simulink model "Roboter_RRP_Sim"  (R2015b)
settings: Solver=ode15s  StartTime=0.0  StopTime=5  RelTol=1e-6  AbsTol=1e-5
InitFcn:
  | set_parameter
StartFcn:
  | set_parameter
StopFcn:
  | Auswertung
undefined symbols (not defined in the file or in its folder): parReg, parSys
settings Model: Creator=andreas  LastModifiedBy=Andreas
settings SolverCC: MaxOrder=3
settings DataIOCC: SaveFormat=Array  SignalLoggingSaveFormat=ModelDataLogs
settings OptimizationCC: ExpressionDepthLimit=2147483647  InitFltsAndDblsToZero=on
settings DebuggingCC: SaveWithParameterizedLinksMsg=none  UnderspecifiedInitializationDetection=Classic  MergeDetectMultiDrivingBlocksExec=none  SignalResolutionControl=TryResolveAllWithWarning  SolverPrmCheckMsg=warning  MultiTaskDSMMsg=warning  MultiTaskCondExecSysMsg=none  FcnCallInpInsideContextMsg=UseLocalSettings  StateNameClashWarn=warning
settings HardwareCC: ProdBitPerPointer=32  ProdLargestAtomicFloat=None  ProdIntDivRoundTo=Undefined  ProdEndianess=Unspecified  ProdWordSize=32  ProdHWDeviceType=32-bit Generic
settings GRTTargetCC: TargetFcnLib=ansi_tfl_tmw.mat  GeneratePreprocessorConditionals=Disable all  CombineOutputUpdateFcns=off  GRTInterface=on
settings ConfigComp: CovModelRefEnable=Off

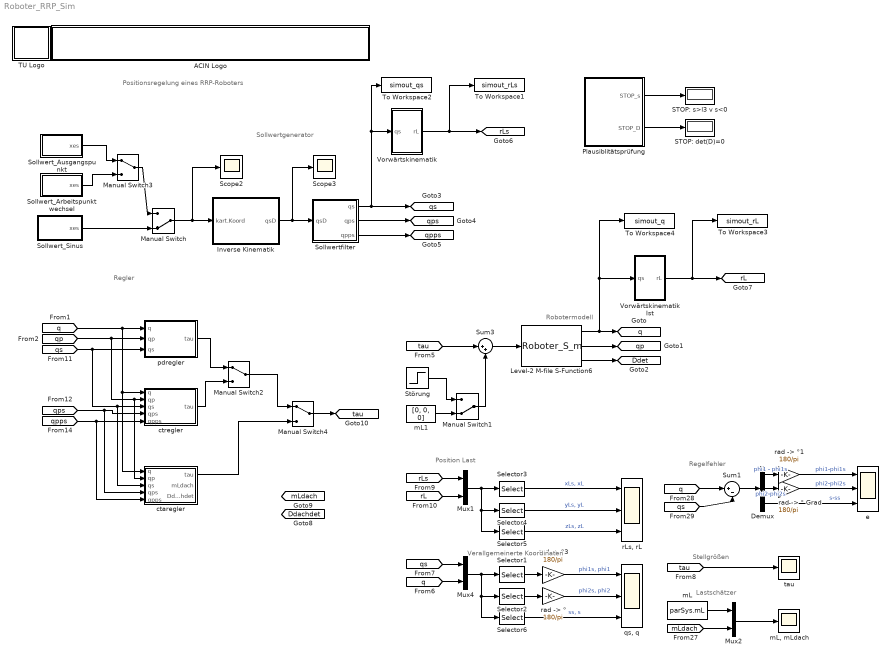
== system Roboter_RRP_Sim ==
  note: Positionsregelung eines RRP-Roboters
  note: Robotermodell
  note: Regler
  note: Sollwertgenerator
  note: Position Last
  note: Verallgemeinerte Koordinaten
  note: Regelfehler
  note: Stellgrößen
  note: Lastschätzer
  ACIN Logo : Subsystem
      mask init:
      | s = get_param(gcb,'UserData');
      mask Display:
      | image(s.logo,[0 0 439 45]);
      | %axis image
  Demux : Demux  Outputs=3
  Inverse Kinematik : Subsystem
  Level-2 M-file S-Function6 : M-S-Function  FunctionName=Roboter_S_m  Parameters=m1,m2,m3,mL,l1,l2,l3,Ixx1,Iyy1,Izz1,Ixx2,Iyy2,Izz2,Ixx3,Iyy3,Izz3,d1,d2,d3,phi10,phi20,s0  mask{m1=parSys.m1, m2=parSys.m2, m3=parSys.m3, mL=parSys.mL, l1=parSys.l1, l2=parSys.l2, l3=parSys.l3, Ixx1=parSys.Ixx1, Iyy1=parSys.Iyy1, Izz1=parSys.Izz1, Ixx2=parSys.Ixx2, Iyy2=parSys.Iyy2, Izz2=parSys.Izz2, Ixx3=parSys.Ixx3, Iyy3=parSys.Iyy3, Izz3=parSys.Izz3, d1=parSys.d1, d2=parSys.d2, d3=parSys.d3, phi10=parSys.phi10, phi20=parSys.phi20, s0=parSys.s0}
      mask prompts: m1 "Masse Stab 1"; m2 "Masse Stab 2"; m3 "Masse Stab 3"; mL "Masse Last"; l1 "Länge Stab 1"; l2 "Länge Stab 2"; l3 "Länge Stab 3"; Ixx1 "Trägheitsmoment x Stab 1"; Iyy1 "Trägheitsmoment y Stab 1"; Izz1 "Trägheitsmoment z Stab 1"; Ixx2 "Trägheitsmoment x Stab 2"; Iyy2 "Trägheitsmoment y Stab 2"; Izz2 "Trägheitsmoment z Stab 2"; Ixx3 "Trägheitsmoment x Stab 3"; Iyy3 "Trägheitsmoment y Stab 3"; Izz3 "Trägheitsmoment z Stab 3"; d1 "Dämpfung Stab 1"; d2 "Dämpfung Stab 2"; d3 "Dämpfung Stab 3"; phi10 "AB phi1"; phi20 "AB phi2"; s0 "AB s"
  Manual Switch : ManualSwitch  CurrentSetting=0
  Manual Switch1 : ManualSwitch  CurrentSetting=0
  Manual Switch2 : ManualSwitch
  Manual Switch3 : ManualSwitch
  Manual Switch4 : ManualSwitch
  Mux1 : Mux  Inputs=2
  Mux2 : Mux  Inputs=2
  Mux4 : Mux  Inputs=2
  Plausiblitätsprüfung : Subsystem
  STOP: det(D)=0 : Display
  STOP: s>l3 v s<0 : Display
  Scope2 : Scope
  Scope3 : Scope
  Selector1 : Selector  InputPortWidth=6  IndexOptions=Index vector (dialog)  Indices=[1 4]  OutputSizes=1
  Selector2 : Selector  InputPortWidth=6  IndexOptions=Index vector (dialog)  Indices=[2 5]  OutputSizes=1
  Selector3 : Selector  InputPortWidth=6  IndexOptions=Index vector (dialog)  Indices=[1 4]  OutputSizes=1
  Selector4 : Selector  InputPortWidth=6  IndexOptions=Index vector (dialog)  Indices=[2 5]  OutputSizes=1
  Selector5 : Selector  InputPortWidth=6  IndexOptions=Index vector (dialog)  Indices=[3 6]  OutputSizes=1
  Selector6 : Selector  InputPortWidth=6  IndexOptions=Index vector (dialog)  Indices=[3 6]  OutputSizes=1
  Sollwert_Arbeitspunktwechsel : Subsystem
  Sollwert_Ausgangspunkt : Subsystem
  Sollwert_Sinus : Subsystem
  Sollwertfilter : Subsystem
  Störung : Step  After=[300, 300, 200]  SampleTime=0
  Sum1 : Sum  Inputs=|+-
  Sum3 : Sum  Inputs=|++
  TU Logo : Subsystem
      mask init:
      | s = get_param(gcb,'UserData');
      mask Display: image(s.logo,[0 0 45 45]);
  To Workspace1 : ToWorkspace  VariableName=simout_rLs  SaveFormat=Structure With Time  SampleTime=-1
  To Workspace2 : ToWorkspace  VariableName=simout_qs  SaveFormat=Structure With Time  SampleTime=-1
  To Workspace3 : ToWorkspace  VariableName=simout_rL  SaveFormat=Structure With Time  SampleTime=-1
  To Workspace4 : ToWorkspace  VariableName=simout_q  SaveFormat=Structure With Time  SampleTime=-1
  Vorwärtskinematik : Subsystem
  Vorwärtskinematik Ist : Subsystem
  ctaregler : MATLAB Function  TreatAsAtomicUnit=on
  ctregler : MATLAB Function  TreatAsAtomicUnit=on
  e : Scope  NumInputPorts=3
  mL : Constant  Value=parSys.mL
  "mL, mLdach" : Scope
  mL1 : Constant  Value=[0, 0, 0]
  pdregler : MATLAB Function  TreatAsAtomicUnit=on
  "qs, q" : Scope  NumInputPorts=3
  "rLs, rL" : Scope  NumInputPorts=3
  "rad -> °" : Gain  Gain=180/pi
  "rad -> ° Grad" : Gain  Gain=180/pi
  "rad -> °1" : Gain  Gain=180/pi
  "rad -> °3" : Gain  Gain=180/pi
  tau : Scope
  tag scope: Ddachdet=global, Ddet=global, mLdach=global, q=global, qp=global, qpps=global, qps=global, qs=global, rL=global, rLs=global, tau=global
  wires:
  Level-2 M-file S-Function6/1 -> [q], Vorwärtskinematik Ist/1(qs), To Workspace4/1
  Level-2 M-file S-Function6/2 -> [qp]
  Inverse Kinematik/1(qsD) -> Scope3/1, Sollwertfilter/1(qsD)
  [tau] -> tau/1
  Vorwärtskinematik Ist/1(rL) -> [rL], To Workspace3/1
  Manual Switch/1 -> Inverse Kinematik/1(kart.Koord), Scope2/1
  Sollwert_Sinus/1(xes) -> Manual Switch/2
  [qs] -> Mux4/1
  [q] -> Mux4/2
  Mux4/1 -> Selector1/1, Selector2/1, Selector6/1
  [rLs] -> Mux1/1
  [rL] -> Mux1/2
  Selector3/1 -> "rLs, rL"/1  "xLs, xL"
  Selector4/1 -> "rLs, rL"/2  "yLs, yL"
  Selector5/1 -> "rLs, rL"/3  "zLs, zL"
  Mux1/1 -> Selector5/1, Selector4/1, Selector3/1
  Manual Switch3/1 -> Manual Switch/1
  Sollwert_Arbeitspunktwechsel/1(xes) -> Manual Switch3/2
  Sollwert_Ausgangspunkt/1(xes) -> Manual Switch3/1
  Plausiblitätsprüfung/1(STOP_s) -> STOP: s>l3 v s<0/1
  Sollwertfilter/1(qs) -> [qs], Vorwärtskinematik/1(qs), To Workspace2/1
  Sollwertfilter/3(qpps) -> [qpps]
  Sollwertfilter/2(qps) -> [qps]
  [q] -> Sum1/1
  Demux/1 -> "rad -> °1"/1  "phi1 - phi1s"
  Demux/2 -> "rad -> ° Grad"/1  "phi2-phi2s"
  Demux/3 -> e/3  "s-ss"
  [qs] -> Sum1/2
  Sum1/1 -> Demux/1
  [tau] -> Sum3/1
  Sum3/1 -> Level-2 M-file S-Function6/1
  Störung/1 -> Manual Switch1/1
  mL1/1 -> Manual Switch1/2
  Manual Switch1/1 -> Sum3/2
  Mux2/1 -> "mL, mLdach"/1
  mL/1 -> Mux2/1
  [mLdach] -> Mux2/2
  Selector1/1 -> "rad -> °3"/1
  Selector2/1 -> "rad -> °"/1
  Selector6/1 -> "qs, q"/3  "ss, s"
  "rad -> °"/1 -> "qs, q"/2  "phi2s, phi2"
  "rad -> °3"/1 -> "qs, q"/1  "phi1s, phi1"
  "rad -> °1"/1 -> e/1  "phi1-phi1s"
  "rad -> ° Grad"/1 -> e/2  "phi2-phi2s"
  Vorwärtskinematik/1(rL) -> [rLs], To Workspace1/1
  Plausiblitätsprüfung/2(STOP_D) -> STOP: det(D)=0/1
  Level-2 M-file S-Function6/3 -> [Ddet]
  [q] -> ctaregler/1(q), ctregler/1(q), pdregler/1(q)
  [qs] -> ctaregler/3(qs), ctregler/3(qs), pdregler/3(qs)
  pdregler/1(tau) -> Manual Switch2/1
  ctregler/1(tau) -> Manual Switch2/2
  [qpps] -> ctaregler/5(qpps), ctregler/5(qpps)
  [qps] -> ctaregler/4(qps), ctregler/4(qps)
  [qp] -> ctaregler/2(qp), ctregler/2(qp), pdregler/2(qp)
  Manual Switch4/1 -> [tau]
  Manual Switch2/1 -> Manual Switch4/1
  ctaregler/1(tau) -> Manual Switch4/2

== system Roboter_RRP_Sim/ACIN Logo ==

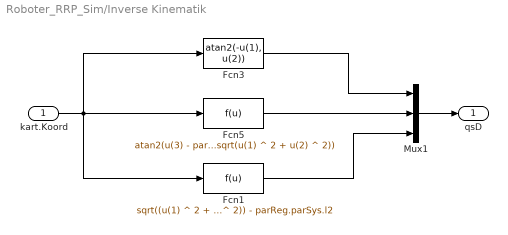
== system Roboter_RRP_Sim/Inverse Kinematik ==
  kart.Koord : Inport
  Fcn1 : Fcn  Expr=sqrt((u(1) ^ 2 + u(2) ^ 2 + u(3) ^ 2 - 2 * u(3) * parReg.parSys.l1 + parReg.parSys.l1 ^ 2)) - parReg.parSys.l2
  Fcn3 : Fcn  Expr=atan2(-u(1), u(2))
  Fcn5 : Fcn  Expr=atan2(u(3) - parReg.parSys.l1, sqrt(u(1) ^ 2 + u(2) ^ 2))
  Mux1 : Mux  Inputs=3
  qsD : Outport
  wires:
  kart.Koord/1 -> Fcn3/1, Fcn1/1, Fcn5/1
  Fcn3/1 -> Mux1/1
  Fcn5/1 -> Mux1/2
  Mux1/1 -> qsD/1
  Fcn1/1 -> Mux1/3

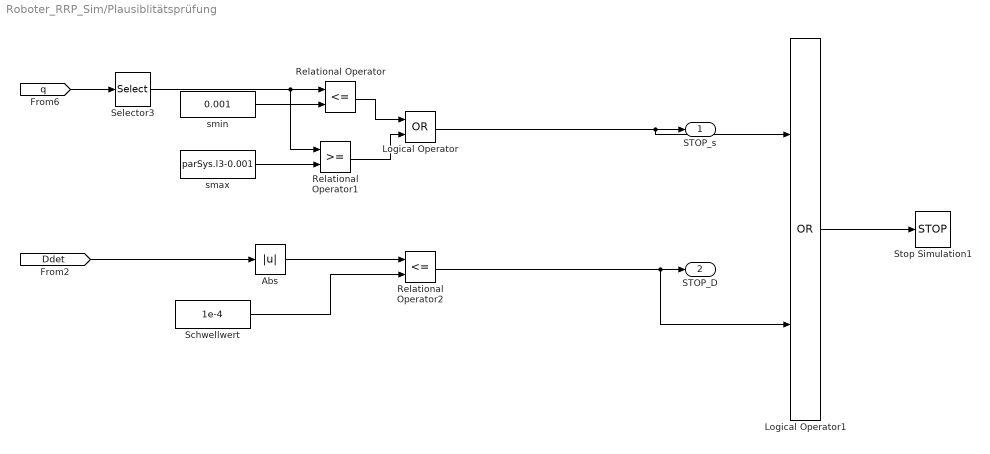
== system Roboter_RRP_Sim/Plausiblitätsprüfung ==
  Abs : Abs
  Logical Operator : Logic  Operator=OR  AllPortsSameDT=off  OutDataTypeStr=boolean
  Logical Operator1 : Logic  Operator=OR  AllPortsSameDT=off  OutDataTypeStr=boolean
  Relational Operator : RelationalOperator  Operator=<=  OutDataTypeStr=boolean
  Relational Operator1 : RelationalOperator  OutDataTypeStr=boolean
  Relational Operator2 : RelationalOperator  Operator=<=  OutDataTypeStr=boolean
  Schwellwert : Constant  Value=1e-4
  Selector3 : Selector  InputPortWidth=3  IndexOptions=Index vector (dialog)  Indices=[3]  OutputSizes=1
  Stop Simulation1 : Stop
  smax : Constant  Value=parSys.l3-0.001
  smin : Constant  Value=0.001
  STOP_s : Outport
  STOP_D : Outport  Port=2
  wires:
  Relational Operator/1 -> Logical Operator/1
  Relational Operator1/1 -> Logical Operator/2
  [q] -> Selector3/1
  Selector3/1 -> Relational Operator/1, Relational Operator1/1
  smin/1 -> Relational Operator/2
  [Ddet] -> Abs/1
  Abs/1 -> Relational Operator2/1
  Schwellwert/1 -> Relational Operator2/2
  Logical Operator1/1 -> Stop Simulation1/1
  smax/1 -> Relational Operator1/2
  Relational Operator2/1 -> STOP_D/1, Logical Operator1/2
  Logical Operator/1 -> STOP_s/1, Logical Operator1/1

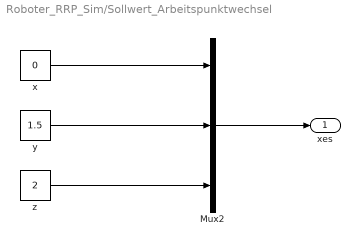
== system Roboter_RRP_Sim/Sollwert_Arbeitspunktwechsel ==
  Mux2 : Mux  Inputs=3
  x : Constant  Value=0
  y : Constant  Value=1.5
  z : Constant  Value=2
  xes : Outport
  wires:
  Mux2/1 -> xes/1
  x/1 -> Mux2/1
  y/1 -> Mux2/2
  z/1 -> Mux2/3

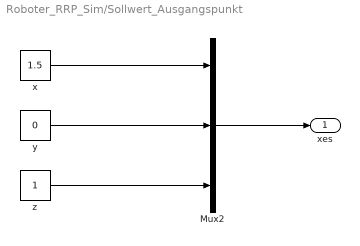
== system Roboter_RRP_Sim/Sollwert_Ausgangspunkt ==
  Mux2 : Mux  Inputs=3
  x : Constant  Value=1.5
  y : Constant  Value=0
  z : Constant
  xes : Outport
  wires:
  z/1 -> Mux2/3
  y/1 -> Mux2/2
  x/1 -> Mux2/1
  Mux2/1 -> xes/1

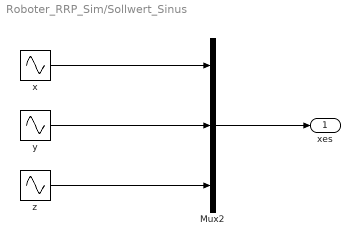
== system Roboter_RRP_Sim/Sollwert_Sinus ==
  Mux2 : Mux  Inputs=3
  x : Sin  Amplitude=1.5  Frequency=2*pi*parReg.traj_fKreis  Phase=pi/2  SampleTime=0
  y : Sin  Amplitude=1.5  Frequency=2*pi*parReg.traj_fKreis  SampleTime=0
  z : Sin  Amplitude=0.5  Bias=1.5  Frequency=2*pi*parReg.traj_fz  Phase=-pi/2  SampleTime=0
  xes : Outport
  wires:
  Mux2/1 -> xes/1
  x/1 -> Mux2/1
  y/1 -> Mux2/2
  z/1 -> Mux2/3

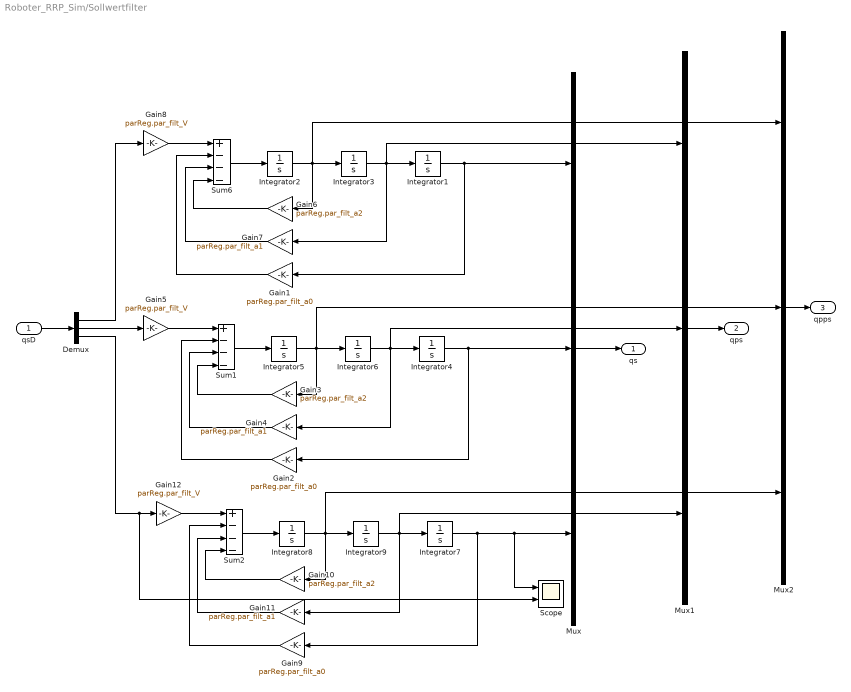
== system Roboter_RRP_Sim/Sollwertfilter ==
  qsD : Inport
  Demux : Demux  Outputs=3
  Gain1 : Gain  Gain=parReg.par_filt_a0  SaturateOnIntegerOverflow=on  OutDataTypeStr=Inherit: Same as input  ParamDataTypeStr=Inherit: Same as input
  Gain10 : Gain  Gain=parReg.par_filt_a2  SaturateOnIntegerOverflow=on  OutDataTypeStr=Inherit: Same as input  ParamDataTypeStr=Inherit: Same as input
  Gain11 : Gain  Gain=parReg.par_filt_a1  SaturateOnIntegerOverflow=on  OutDataTypeStr=Inherit: Same as input  ParamDataTypeStr=Inherit: Same as input
  Gain12 : Gain  Gain=parReg.par_filt_V  SaturateOnIntegerOverflow=on  OutDataTypeStr=Inherit: Same as input  ParamDataTypeStr=Inherit: Same as input
  Gain2 : Gain  Gain=parReg.par_filt_a0  SaturateOnIntegerOverflow=on  OutDataTypeStr=Inherit: Same as input  ParamDataTypeStr=Inherit: Same as input
  Gain3 : Gain  Gain=parReg.par_filt_a2  SaturateOnIntegerOverflow=on  OutDataTypeStr=Inherit: Same as input  ParamDataTypeStr=Inherit: Same as input
  Gain4 : Gain  Gain=parReg.par_filt_a1  SaturateOnIntegerOverflow=on  OutDataTypeStr=Inherit: Same as input  ParamDataTypeStr=Inherit: Same as input
  Gain5 : Gain  Gain=parReg.par_filt_V  SaturateOnIntegerOverflow=on  OutDataTypeStr=Inherit: Same as input  ParamDataTypeStr=Inherit: Same as input
  Gain6 : Gain  Gain=parReg.par_filt_a2  SaturateOnIntegerOverflow=on  OutDataTypeStr=Inherit: Same as input  ParamDataTypeStr=Inherit: Same as input
  Gain7 : Gain  Gain=parReg.par_filt_a1  SaturateOnIntegerOverflow=on  OutDataTypeStr=Inherit: Same as input  ParamDataTypeStr=Inherit: Same as input
  Gain8 : Gain  Gain=parReg.par_filt_V  SaturateOnIntegerOverflow=on  OutDataTypeStr=Inherit: Same as input  ParamDataTypeStr=Inherit: Same as input
  Gain9 : Gain  Gain=parReg.par_filt_a0  SaturateOnIntegerOverflow=on  OutDataTypeStr=Inherit: Same as input  ParamDataTypeStr=Inherit: Same as input
  Integrator1 : Integrator  InitialCondition=parReg.traj_phi10
  Integrator{2..3,5..6,8..9} (6 alike) : Integrator
  Integrator4 : Integrator  InitialCondition=parReg.traj_phi20
  Integrator7 : Integrator  InitialCondition=parReg.traj_s0
  Mux : Mux  Inputs=3
  Mux1 : Mux  Inputs=3
  Mux2 : Mux  Inputs=3
  Scope : Scope  NumInputPorts=2
  Sum1 : Sum  Inputs=+---  SaturateOnIntegerOverflow=on  InputSameDT=on  OutDataTypeStr=Inherit: Same as first input
  Sum2 : Sum  Inputs=+---  SaturateOnIntegerOverflow=on  InputSameDT=on  OutDataTypeStr=Inherit: Same as first input
  Sum6 : Sum  Inputs=+---  SaturateOnIntegerOverflow=on  InputSameDT=on  OutDataTypeStr=Inherit: Same as first input
  qs : Outport
  qps : Outport  Port=2
  qpps : Outport  Port=3
  wires:
  Mux/1 -> qs/1
  qsD/1 -> Demux/1
  Demux/1 -> Gain8/1
  Sum6/1 -> Integrator2/1
  Gain8/1 -> Sum6/1
  Integrator3/1 -> Integrator1/1, Gain7/1, Mux1/1
  Integrator2/1 -> Integrator3/1, Gain6/1, Mux2/1
  Integrator1/1 -> Gain1/1, Mux/1
  Gain6/1 -> Sum6/4
  Gain7/1 -> Sum6/3
  Gain1/1 -> Sum6/2
  Sum1/1 -> Integrator5/1
  Gain5/1 -> Sum1/1
  Integrator6/1 -> Gain4/1, Integrator4/1, Mux1/2
  Integrator5/1 -> Gain3/1, Integrator6/1, Mux2/2
  Integrator4/1 -> Gain2/1, Mux/2
  Gain3/1 -> Sum1/4
  Gain4/1 -> Sum1/3
  Gain2/1 -> Sum1/2
  Demux/2 -> Gain5/1
  Sum2/1 -> Integrator8/1
  Gain12/1 -> Sum2/1
  Integrator9/1 -> Integrator7/1, Gain11/1, Mux1/3
  Integrator8/1 -> Integrator9/1, Gain10/1, Mux2/3
  Integrator7/1 -> Gain9/1, Mux/3, Scope/1
  Gain10/1 -> Sum2/4
  Gain11/1 -> Sum2/3
  Gain9/1 -> Sum2/2
  Demux/3 -> Gain12/1, Scope/2
  Mux1/1 -> qps/1
  Mux2/1 -> qpps/1

== system Roboter_RRP_Sim/TU Logo ==

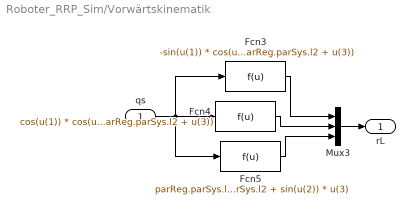
== system Roboter_RRP_Sim/Vorwärtskinematik ==
  qs : Inport
  Fcn3 : Fcn  Expr=-sin(u(1)) * cos(u(2)) * (parReg.parSys.l2 + u(3))
  Fcn4 : Fcn  Expr=cos(u(1)) * cos(u(2)) * (parReg.parSys.l2 + u(3))
  Fcn5 : Fcn  Expr=parReg.parSys.l1 + sin(u(2)) * parReg.parSys.l2 + sin(u(2)) * u(3)
  Mux3 : Mux  Inputs=3
  rL : Outport
  wires:
  Fcn3/1 -> Mux3/1
  Fcn4/1 -> Mux3/2
  Fcn5/1 -> Mux3/3
  qs/1 -> Fcn5/1, Fcn4/1, Fcn3/1
  Mux3/1 -> rL/1

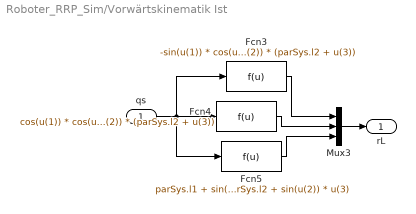
== system Roboter_RRP_Sim/Vorwärtskinematik Ist ==
  qs : Inport
  Fcn3 : Fcn  Expr=-sin(u(1)) * cos(u(2)) * (parSys.l2 + u(3))
  Fcn4 : Fcn  Expr=cos(u(1)) * cos(u(2)) * (parSys.l2 + u(3))
  Fcn5 : Fcn  Expr=parSys.l1 + sin(u(2)) * parSys.l2 + sin(u(2)) * u(3)
  Mux3 : Mux  Inputs=3
  rL : Outport
  wires:
  Mux3/1 -> rL/1
  qs/1 -> Fcn3/1, Fcn4/1, Fcn5/1
  Fcn5/1 -> Mux3/3
  Fcn4/1 -> Mux3/2
  Fcn3/1 -> Mux3/1

== matlab function Roboter_RRP_Sim/ctregler ==
  settings: updateMethod=DISCRETE  sampleTime=parReg.CT.Ts
  data: q input; tau output; qp input; qs input; qps input; qpps input; parSys parameter; parReg parameter
function tau = ctregler(q,qp,qs,qps,qpps,parSys, parReg)

m1 = parSys.m1;
m2 = parSys.m2;
m3 = parSys.m3;
mL = parReg.parSys.mL;
l1 = parSys.l1;
l2 = parSys.l2;
l3 = parSys.l3;
Ixx1 = parSys.Ixx1;
Iyy1 = parSys.Iyy1;
Izz1 = parSys.Izz1;
Ixx2 = parSys.Ixx2;
Iyy2 = parSys.Iyy2;
Izz2 = parSys.Izz2;
Ixx3 = parSys.Ixx3;
Iyy3 = parSys.Iyy3;
Izz3 = parSys.Izz3;
d1 = parSys.d1;
d2 = parSys.d2;
d3 = parSys.d3;
delta_phi10 = parSys.delta_phi10;    
delta_phi20 = parSys.delta_phi20;
delta_s0 = parSys.delta_s0;   
phi10 = parSys.phi10;
phi20 = parSys.phi20; 
s0 = parSys.s0; 
g=9.81;

phi1 = q(1);
phi2 = q(2);
s = q(3);
phi1p = qp(1);
phi2p = qp(2);
sp = qp(3);

gg = [0 (m2 * l2 + 2 * m3 * l2 + 2 * m3 * s - m3 * l3 + 2 * mL * l2 + 2 * s * mL) * cos(phi2) * g / 0.2e1 (m3 + mL) * sin(phi2) * g];
DD = [m2 * cos(phi2) ^ 2 * l2 ^ 2 / 0.4e1 + m3 * cos(phi2) ^ 2 * l2 ^ 2 + 0.2e1 * m3 * cos(phi2) ^ 2 * l2 * s - m3 * cos(phi2) ^ 2 * l2 * l3 + m3 * cos(phi2) ^ 2 * s ^ 2 - m3 * cos(phi2) ^ 2 * s * l3 + m3 * cos(phi2) ^ 2 * l3 ^ 2 / 0.4e1 + mL * cos(phi2) ^ 2 * l2 ^ 2 + 0.2e1 * mL * cos(phi2) ^ 2 * l2 * s + mL * cos(phi2) ^ 2 * s ^ 2 + Izz1 + cos(phi2) ^ 2 * Izz2 + Iyy2 - Iyy2 * cos(phi2) ^ 2 + cos(phi2) ^ 2 * Izz3 + Iyy3 - Iyy3 * cos(phi2) ^ 2 0 0; 0 m2 * l2 ^ 2 / 0.4e1 + m3 * l2 ^ 2 + 0.2e1 * m3 * l2 * s - m3 * l2 * l3 + m3 * s ^ 2 - m3 * s * l3 + m3 * l3 ^ 2 / 0.4e1 + mL * l2 ^ 2 + 0.2e1 * mL * l2 * s + mL * s ^ 2 + Ixx2 + Ixx3 0; 0 0 m3 + mL;];
CC = [cos(phi2) * (-sin(phi2) * phi2p * m2 * l2 ^ 2 - 0.4e1 * sin(phi2) * phi2p * m3 * l2 ^ 2 - 0.4e1 * sin(phi2) * phi2p * mL * l2 ^ 2 + 0.4e1 * sin(phi2) * phi2p * m3 * l2 * l3 - 0.8e1 * sin(phi2) * phi2p * m3 * l2 * s - 0.8e1 * sin(phi2) * phi2p * mL * l2 * s - 0.4e1 * sin(phi2) * phi2p * m3 * s ^ 2 + 0.4e1 * sin(phi2) * phi2p * m3 * s * l3 - sin(phi2) * phi2p * m3 * l3 ^ 2 + 0.4e1 * sin(phi2) * phi2p * Iyy3 - 0.4e1 * sin(phi2) * phi2p * mL * s ^ 2 - 0.4e1 * sin(phi2) * phi2p * Izz2 + 0.4e1 * sin(phi2) * phi2p * Iyy2 - 0.4e1 * sin(phi2) * phi2p * Izz3 + 0.4e1 * cos(phi2) * sp * m3 * l2 + 0.4e1 * cos(phi2) * sp * mL * l2 + 0.4e1 * cos(phi2) * sp * m3 * s - 0.2e1 * cos(phi2) * sp * m3 * l3 + 0.4e1 * cos(phi2) * sp * s * mL) / 0.4e1 (-0.4e1 * m3 * l2 ^ 2 + 0.4e1 * m3 * l2 * l3 - m2 * l2 ^ 2 + 0.4e1 * m3 * s * l3 - 0.4e1 * mL * l2 ^ 2 - 0.4e1 * m3 * s ^ 2 - 0.4e1 * mL * s ^ 2 - m3 * l3 ^ 2 - 0.4e1 * Izz2 - 0.8e1 * mL * l2 * s + 0.4e1 * Iyy2 - 0.4e1 * Izz3 - 0.8e1 * m3 * l2 * s + 0.4e1 * Iyy3) * cos(phi2) * sin(phi2) * phi1p / 0.4e1 (0.2e1 * m3 * l2 + 0.2e1 * m3 * s - m3 * l3 + 0.2e1 * mL * l2 + 0.2e1 * s * mL) * cos(phi2) ^ 2 * phi1p / 0.2e1; -(-0.4e1 * m3 * l2 ^ 2 + 0.4e1 * m3 * l2 * l3 - m2 * l2 ^ 2 + 0.4e1 * m3 * s * l3 - 0.4e1 * mL * l2 ^ 2 - 0.4e1 * m3 * s ^ 2 - 0.4e1 * mL * s ^ 2 - m3 * l3 ^ 2 - 0.4e1 * Izz2 - 0.8e1 * mL * l2 * s + 0.4e1 * Iyy2 - 0.4e1 * Izz3 - 0.8e1 * m3 * l2 * s + 0.4e1 * Iyy3) * cos(phi2) * sin(phi2) * phi1p / 0.4e1 (0.2e1 * m3 * l2 + 0.2e1 * m3 * s - m3 * l3 + 0.2e1 * mL * l2 + 0.2e1 * s * mL) * sp / 0.2e1 (0.2e1 * m3 * l2 + 0.2e1 * m3 * s - m3 * l3 + 0.2e1 * mL * l2 + 0.2e1 * s * mL) * phi2p / 0.2e1; -(0.2e1 * m3 * l2 + 0.2e1 * m3 * s - m3 * l3 + 0.2e1 * mL * l2 + 0.2e1 * s * mL) * cos(phi2) ^ 2 * phi1p / 0.2e1 -(0.2e1 * m3 * l2 + 0.2e1 * m3 * s - m3 * l3 + 0.2e1 * mL * l2 + 0.2e1 * s * mL) * phi2p / 0.2e1 0;];
rr = [d1 * phi1p d2 * phi2p d3 * sp];

v = qpps - parReg.CT.K0*(q-qs)-parReg.CT.K1*(qp-qps);
tau = DD*v+CC*qp+gg'+rr';

== matlab function Roboter_RRP_Sim/pdregler ==
  settings: updateMethod=DISCRETE  sampleTime=parReg.PD.Ts
  data: q input; tau output; qp input; qs input; parSys parameter; parReg parameter
function tau = pdregler(q,qp,qs, parSys, parReg)

m1 = parSys.m1;
m2 = parSys.m2;
m3 = parSys.m3;
mL = parSys.mL;
l1 = parSys.l1;
l2 = parSys.l2;
l3 = parSys.l3;
Ixx1 = parSys.Ixx1;
Iyy1 = parSys.Iyy1;
Izz1 = parSys.Izz1;
Ixx2 = parSys.Ixx2;
Iyy2 = parSys.Iyy2;
Izz2 = parSys.Izz2;
Ixx3 = parSys.Ixx3;
Iyy3 = parSys.Iyy3;
Izz3 = parSys.Izz3;
d1 = parSys.d1;
d2 = parSys.d2;
d3 = parSys.d3;
delta_phi10 = parSys.delta_phi10;    
delta_phi20 = parSys.delta_phi20;
delta_s0 = parSys.delta_s0;   
phi10 = parSys.phi10;
phi20 = parSys.phi20; 
s0 = parSys.s0; 
g=9.81;

phi1 = q(1);
phi2 = q(2);
s = q(3);

gg = [0 (m2 * l2 + 2 * m3 * l2 + 2 * m3 * s - m3 * l3 + 2 * mL * l2 + 2 * s * mL) * cos(phi2) * g / 0.2e1 (m3 + mL) * sin(phi2) * g];

tau = -parReg.PD.KP*(q-qs)-parReg.PD.KD*qp+gg';

== matlab function Roboter_RRP_Sim/ctaregler ==
  settings: updateMethod=DISCRETE  sampleTime=5e-3
  data: q input; tau output; qp input; qs input; qps input; qpps input; parSys parameter; parReg parameter; mLdach output; Ddachdet output
function [tau,mLdach,Ddachdet] = ctaregler(q,qp,qs,qps,qpps,parSys, parReg)
persistent pdach

if isempty(pdach) pdach = parReg.parSys.mL; end
m1 = parSys.m1;
m2 = parSys.m2;
m3 = parSys.m3;
mL = parReg.parSys.mL;
l1 = parSys.l1;
l2 = parSys.l2;
l3 = parSys.l3;
Ixx1 = parSys.Ixx1;
Iyy1 = parSys.Iyy1;
Izz1 = parSys.Izz1;
Ixx2 = parSys.Ixx2;
Iyy2 = parSys.Iyy2;
Izz2 = parSys.Izz2;
Ixx3 = parSys.Ixx3;
Iyy3 = parSys.Iyy3;
Izz3 = parSys.Izz3;
d1 = parSys.d1;
d2 = parSys.d2;
d3 = parSys.d3;
delta_phi10 = parSys.delta_phi10;    
delta_phi20 = parSys.delta_phi20;
delta_s0 = parSys.delta_s0;   
phi10 = parSys.phi10;
phi20 = parSys.phi20; 
s0 = parSys.s0; 
g=9.81;
phi1 = q(1);
phi2 = q(2);
s = q(3);
phi1p = qp(1);
phi2p = qp(2);
sp = qp(3);

pdach = pdach + parReg.CTA.Ts*(-parReg.CTA.Gamma^(-1)*phi'*parReg.CTA.B'*parReg.CTA.P*[q-qs;qp-qps]);
gg = [0 (m2 * l2 + 2 * m3 * l2 + 2 * m3 * s - m3 * l3 + 2 * pdach * l2 + 2 * s * pdach) * cos(phi2) * g / 0.2e1 (m3 + pdach) * sin(phi2) * g];
DD = [m2 * cos(phi2) ^ 2 * l2 ^ 2 / 0.4e1 + m3 * cos(phi2) ^ 2 * l2 ^ 2 + 0.2e1 * m3 * cos(phi2) ^ 2 * l2 * s - m3 * cos(phi2) ^ 2 * l2 * l3 + m3 * cos(phi2) ^ 2 * s ^ 2 - m3 * cos(phi2) ^ 2 * s * l3 + m3 * cos(phi2) ^ 2 * l3 ^ 2 / 0.4e1 + pdach * cos(phi2) ^ 2 * l2 ^ 2 + 0.2e1 * pdach * cos(phi2) ^ 2 * l2 * s + pdach * cos(phi2) ^ 2 * s ^ 2 + Izz1 + cos(phi2) ^ 2 * Izz2 + Iyy2 - Iyy2 * cos(phi2) ^ 2 + cos(phi2) ^ 2 * Izz3 + Iyy3 - Iyy3 * cos(phi2) ^ 2 0 0; 0 m2 * l2 ^ 2 / 0.4e1 + m3 * l2 ^ 2 + 0.2e1 * m3 * l2 * s - m3 * l2 * l3 + m3 * s ^ 2 - m3 * s * l3 + m3 * l3 ^ 2 / 0.4e1 + pdach * l2 ^ 2 + 0.2e1 * pdach * l2 * s + pdach * s ^ 2 + Ixx2 + Ixx3 0; 0 0 m3 + pdach;];
CC = [cos(phi2) * (-sin(phi2) * phi2p * m2 * l2 ^ 2 - 0.4e1 * sin(phi2) * phi2p * m3 * l2 ^ 2 - 0.4e1 * sin(phi2) * phi2p * pdach * l2 ^ 2 + 0.4e1 * sin(phi2) * phi2p * m3 * l2 * l3 - 0.8e1 * sin(phi2) * phi2p * m3 * l2 * s - 0.8e1 * sin(phi2) * phi2p * pdach * l2 * s - 0.4e1 * sin(phi2) * phi2p * m3 * s ^ 2 + 0.4e1 * sin(phi2) * phi2p * m3 * s * l3 - sin(phi2) * phi2p * m3 * l3 ^ 2 + 0.4e1 * sin(phi2) * phi2p * Iyy3 - 0.4e1 * sin(phi2) * phi2p * pdach * s ^ 2 - 0.4e1 * sin(phi2) * phi2p * Izz2 + 0.4e1 * sin(phi2) * phi2p * Iyy2 - 0.4e1 * sin(phi2) * phi2p * Izz3 + 0.4e1 * cos(phi2) * sp * m3 * l2 + 0.4e1 * cos(phi2) * sp * pdach * l2 + 0.4e1 * cos(phi2) * sp * m3 * s - 0.2e1 * cos(phi2) * sp * m3 * l3 + 0.4e1 * cos(phi2) * sp * s * pdach) / 0.4e1 (-0.4e1 * m3 * l2 ^ 2 + 0.4e1 * m3 * l2 * l3 - m2 * l2 ^ 2 + 0.4e1 * m3 * s * l3 - 0.4e1 * pdach * l2 ^ 2 - 0.4e1 * m3 * s ^ 2 - 0.4e1 * pdach * s ^ 2 - m3 * l3 ^ 2 - 0.4e1 * Izz2 - 0.8e1 * pdach * l2 * s + 0.4e1 * Iyy2 - 0.4e1 * Izz3 - 0.8e1 * m3 * l2 * s + 0.4e1 * Iyy3) * cos(phi2) * sin(phi2) * phi1p / 0.4e1 (0.2e1 * m3 * l2 + 0.2e1 * m3 * s - m3 * l3 + 0.2e1 * pdach * l2 + 0.2e1 * s * pdach) * cos(phi2) ^ 2 * phi1p / 0.2e1; -(-0.4e1 * m3 * l2 ^ 2 + 0.4e1 * m3 * l2 * l3 - m2 * l2 ^ 2 + 0.4e1 * m3 * s * l3 - 0.4e1 * pdach * l2 ^ 2 - 0.4e1 * m3 * s ^ 2 - 0.4e1 * pdach * s ^ 2 - m3 * l3 ^ 2 - 0.4e1 * Izz2 - 0.8e1 * pdach * l2 * s + 0.4e1 * Iyy2 - 0.4e1 * Izz3 - 0.8e1 * m3 * l2 * s + 0.4e1 * Iyy3) * cos(phi2) * sin(phi2) * phi1p / 0.4e1 (0.2e1 * m3 * l2 + 0.2e1 * m3 * s - m3 * l3 + 0.2e1 * pdach * l2 + 0.2e1 * s * pdach) * sp / 0.2e1 (0.2e1 * m3 * l2 + 0.2e1 * m3 * s - m3 * l3 + 0.2e1 * pdach * l2 + 0.2e1 * s * pdach) * phi2p / 0.2e1; -(0.2e1 * m3 * l2 + 0.2e1 * m3 * s - m3 * l3 + 0.2e1 * pdach * l2 + 0.2e1 * s * pdach) * cos(phi2) ^ 2 * phi1p / 0.2e1 -(0.2e1 * m3 * l2 + 0.2e1 * m3 * s - m3 * l3 + 0.2e1 * pdach * l2 + 0.2e1 * s * pdach) * phi2p / 0.2e1 0;];
rr = [d1 * phi1p d2 * phi2p d3 * sp];

v = qpps - parReg.CT.K0*(q-qs)-parReg.CT.K1*(qp-qps);
tau = DD*v+CC*qp+gg'+rr';

mLdach = pdach;
end
